simulink model "Linearization"  (R2022a)
settings: Solver=VariableStepAuto  StartTime=0.0  StopTime=100  RelTol=1e-3
undefined symbols (not defined in the file): Aactuator, ac, AeroCoeff, ControlAllocation, DUmax, DUmin, EngineTable, F, fcs, ft, g, hground, IC, kg, LandingGear, Light, LPmethod, m, MIL, Mode_deflection_aileron, Mode_deflection_elevator, Mode_deflection_rudder, Mode_deflection_TVC_y, Mode_deflection_TVC_z, N, Ninv_2nozzle, Ninv_no_nozzle, PIController, s, Sensor, slug, state0, sysID_DAQ, sysID_OBES, Umax_2nozzle, Umax_no_nozzle, Umin_2nozzle, Umin_no_nozzle, WMM2020
libraries: aerolibconvert2 x19, slpidlib x6, simulink x6, sharedutil x4, aerolibatmos2 x3, aerolibwind2 x3, aerolibbdyn x3, aerolibgravity2 x2, sharedtransform x1
(part 2 of 9)

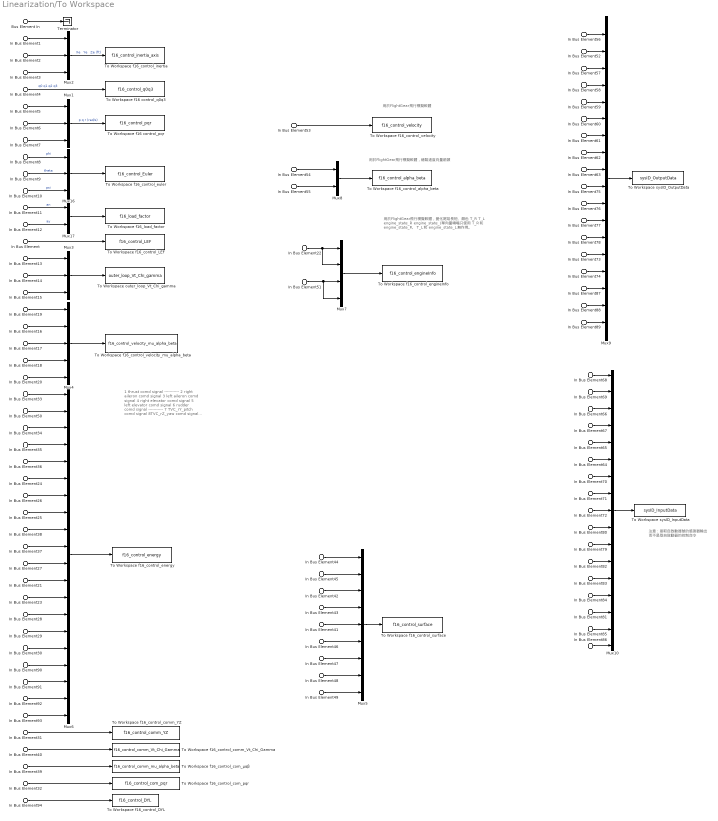
== system Linearization/To Workspace ==
  note: 1 thrust comd signal
      | -----------
      | 2 right aileron comd signal
      | 3 left aileron comd signal
      | 4 right elevator comd signal
      | 5 left elevator comd signal
      | 6 rudder comd signal
      | -----------
      | 7 TVC_rY_pitch comd signal
      | 8TVC_rZ_yaw comd signal
      | 9 TVC_lY_pitch comd signal
      | 10TVC_lZ_yaw comd signal
      |
      | 11 thrust signal
      | -----------
      | 12 right aileron signal
      | 13 left aileron signal
      | 14 right elevator signal
      | 15 left elevator signal
      | 16 rudder signal
      | -----------
      | 17 TVC_rY_pitch signal
      | 18 TVC_rZ_yaw signal
      | 19 TVC_lY_pitch signal
      | 20 TVC_lZ_yaw signal
  note: 用於FlightGear飛行模擬軟體
  note: 用於FlightGear飛行模擬軟體，繪製速度向量箭頭
  note: 用於FlightGear飛行模擬軟體，變化尾焰長短、顏色
      | T_R
      | T_L
      | engine_state_R
      | engine_state_L
      |
      | 單向量噴嘴只使用 T_R 和 engine_state_R。
      | T_L 和 engine_state_L 無作用。
  note: 注意：是取自致動器號的感測器輸出
      | 而不是取自致動器的控制命令
  In Bus Element1 : Inport  PortName=PlantData  Element=npos
  In Bus Element2 : Inport  PortName=PlantData  Element=epos
  In Bus Element3 : Inport  PortName=PlantData  Element=altitude
  In Bus Element4 : Inport  PortName=PlantData  Element=q0q1q2q3
  In Bus Element5 : Inport  PortName=PlantData  Element=p
  In Bus Element61 : Inport  PortName=PlantData  Element=p
  In Bus Element6 : Inport  PortName=PlantData  Element=q
  In Bus Element62 : Inport  PortName=PlantData  Element=q
  In Bus Element7 : Inport  PortName=PlantData  Element=r
  In Bus Element63 : Inport  PortName=PlantData  Element=r
  In Bus Element8 : Inport  PortName=PlantData  Element=phi
  In Bus Element58 : Inport  PortName=PlantData  Element=phi
  In Bus Element9 : Inport  PortName=PlantData  Element=theta
  In Bus Element59 : Inport  PortName=PlantData  Element=theta
  In Bus Element10 : Inport  PortName=PlantData  Element=psi
  In Bus Element60 : Inport  PortName=PlantData  Element=psi
  In Bus Element11 : Inport  PortName=PlantData  Element=an
  In Bus Element12 : Inport  PortName=PlantData  Element=ay
  In Bus Element : Inport  PortName=PlantData  Element=AeroActBus.LEF_deg
  In Bus Element80 : Inport  PortName=PlantData  Element=AeroActBus.LEF_deg
  In Bus Element30 : Inport  PortName=PlantData  Element=AeroActBus.Rudder_deg
  In Bus Element41 : Inport  PortName=PlantData  Element=AeroActBus.Rudder_deg
  In Bus Element65 : Inport  PortName=PlantData  Element=AeroActBus.Rudder_deg
  In Bus Element21 : Inport  PortName=PlantData  Element=AeroActBus.right Aileron_deg
  In Bus Element42 : Inport  PortName=PlantData  Element=AeroActBus.right Aileron_deg
  In Bus Element66 : Inport  PortName=PlantData  Element=AeroActBus.right Aileron_deg
  In Bus Element23 : Inport  PortName=PlantData  Element=AeroActBus.left Aileron_deg
  In Bus Element43 : Inport  PortName=PlantData  Element=AeroActBus.left Aileron_deg
  In Bus Element67 : Inport  PortName=PlantData  Element=AeroActBus.left Aileron_deg
  In Bus Element28 : Inport  PortName=PlantData  Element=AeroActBus.right Elevator_deg
  In Bus Element44 : Inport  PortName=PlantData  Element=AeroActBus.right Elevator_deg
  In Bus Element68 : Inport  PortName=PlantData  Element=AeroActBus.right Elevator_deg
  In Bus Element29 : Inport  PortName=PlantData  Element=AeroActBus.left Elevator_deg
  In Bus Element45 : Inport  PortName=PlantData  Element=AeroActBus.left Elevator_deg
  In Bus Element69 : Inport  PortName=PlantData  Element=AeroActBus.left Elevator_deg
  In Bus Element79 : Inport  PortName=PlantData  Element=AeroActBus.SB_deg
  In Bus Element{13,19,53,56} (4 alike) : Inport  PortName=PlantData  Element=Vt
  In Bus Element14 : Inport  PortName=PlantData  Element=chi
  In Bus Element88 : Inport  PortName=PlantData  Element=chi
  In Bus Element15 : Inport  PortName=PlantData  Element=gamma
  In Bus Element20 : Inport  PortName=PlantData  Element=gamma
  In Bus Element89 : Inport  PortName=PlantData  Element=gamma
  In Bus Element16 : Inport  PortName=PlantData  Element=alpha
  In Bus Element54 : Inport  PortName=PlantData  Element=alpha
  In Bus Element52 : Inport  PortName=PlantData  Element=alpha
  In Bus Element17 : Inport  PortName=PlantData  Element=beta
  In Bus Element55 : Inport  PortName=PlantData  Element=beta
  In Bus Element57 : Inport  PortName=PlantData  Element=beta
  In Bus Element18 : Inport  PortName=PlantData  Element=mu
  In Bus Element87 : Inport  PortName=PlantData  Element=mu
  In Bus Element33 : Inport  PortName=PlantData  Element=fadec_cmd.thrust
  In Bus Element25 : Inport  PortName=PlantData  Element=fadec_cmd.TVC_rz
  In Bus Element26 : Inport  PortName=PlantData  Element=fadec_cmd.TVC_ry
  In Bus Element37 : Inport  PortName=PlantData  Element=fadec_cmd.TVC_lz
  In Bus Element38 : Inport  PortName=PlantData  Element=fadec_cmd.TVC_ly
  In Bus Element24 : Inport  PortName=PlantData  Element=fcs_cmd.rudder
  In Bus Element34 : Inport  PortName=PlantData  Element=fcs_cmd.left aileron
  In Bus Element35 : Inport  PortName=PlantData  Element=fcs_cmd.right elevator
  In Bus Element36 : Inport  PortName=PlantData  Element=fcs_cmd.left elevator
  In Bus Element50 : Inport  PortName=PlantData  Element=fcs_cmd.right aileron
  In Bus Element27 : Inport  PortName=PlantData  Element=PropBus.T
  In Bus Element22 : Inport  PortName=PlantData  Element=PropBus.T
  In Bus Element51 : Inport  PortName=PlantData  Element=PropBus.engine_state
  In Bus Element82 : Inport  PortName=PlantData  Element=PropBus.Tx
  In Bus Element83 : Inport  PortName=PlantData  Element=PropBus.Ty
  In Bus Element84 : Inport  PortName=PlantData  Element=PropBus.Tz
  In Bus Element73 : Inport  PortName=PlantData  Element=ay_offset
  In Bus Element74 : Inport  PortName=PlantData  Element=az_offset
  In Bus Element75 : Inport  PortName=PlantData  Element=p_dot
  In Bus Element76 : Inport  PortName=PlantData  Element=q_dot
  In Bus Element77 : Inport  PortName=PlantData  Element=r_dot
  In Bus Element85 : Inport  PortName=PlantData  Element=f
  In Bus Element86 : Inport  PortName=PlantData  Element=N
  In Bus Element90 : Inport  PortName=PlantData  Element=PropActBus.TVC_ry_pitch_deg
  In Bus Element46 : Inport  PortName=PlantData  Element=PropActBus.TVC_ry_pitch_deg
  In Bus Element64 : Inport  PortName=PlantData  Element=PropActBus.TVC_ry_pitch_deg
  In Bus Element91 : Inport  PortName=PlantData  Element=PropActBus.TVC_rz_yaw_deg
  In Bus Element47 : Inport  PortName=PlantData  Element=PropActBus.TVC_rz_yaw_deg
  In Bus Element70 : Inport  PortName=PlantData  Element=PropActBus.TVC_rz_yaw_deg
  In Bus Element92 : Inport  PortName=PlantData  Element=PropActBus.TVC_ly_pitch_deg
  In Bus Element48 : Inport  PortName=PlantData  Element=PropActBus.TVC_ly_pitch_deg
  In Bus Element71 : Inport  PortName=PlantData  Element=PropActBus.TVC_ly_pitch_deg
  In Bus Element93 : Inport  PortName=PlantData  Element=PropActBus.TVC_lz_yaw_deg
  In Bus Element49 : Inport  PortName=PlantData  Element=PropActBus.TVC_lz_yaw_deg
  In Bus Element72 : Inport  PortName=PlantData  Element=PropActBus.TVC_lz_yaw_deg
  In Bus Element78 : Inport  PortName=PlantData  Element=ax_offset
  In Bus Element32 : Inport  PortName=PlantData  Element=LogDataBus.cmd_pqr
  In Bus Element39 : Inport  PortName=PlantData  Element=LogDataBus.cmd_mu_alpha_beta
  In Bus Element31 : Inport  PortName=PlantData  Element=LogDataBus.cmd_yz
  In Bus Element40 : Inport  PortName=PlantData  Element=LogDataBus.cmd_Vt_chi_gamma
  In Bus Element94 : Inport  PortName=PlantData  Element=LogDataBus.drag_sideForce_lift
  Bus Element In : Inport  Port=2  PortName=EnvData
  In Bus Element81 : Inport  Port=2  PortName=EnvData  Element=AirDensity
  Mux{1..3,16} (4 alike) : Mux  Inputs=3
  Mux10 : Mux  Inputs=17
  Mux17 : Mux  Inputs=2
  Mux4 : Mux  Inputs=5
  Mux5 : Mux  Inputs=9
  Mux6 : Mux  Inputs=20
  Mux7 : Mux
  Mux8 : Mux  Inputs=2
  Mux9 : Mux  Inputs=18
  Terminator : Terminator
  To Workspace f16 control_pqr : ToWorkspace  VariableName=f16_control_pqr  SaveFormat=Timeseries  SampleTime=-1
  To Workspace f16 control_q0q3 : ToWorkspace  VariableName=f16_control_q0q3  SaveFormat=Timeseries  SampleTime=-1
  To Workspace f16_control_DYL : ToWorkspace  VariableName=f16_control_DYL  SaveFormat=Timeseries  SampleTime=-1
  To Workspace f16_control_LEF : ToWorkspace  VariableName=f16_control_LEF  SaveFormat=Timeseries  SampleTime=-1
  To Workspace f16_control_alpha_beta : ToWorkspace  VariableName=f16_control_alpha_beta  SaveFormat=Timeseries  SampleTime=-1
  To Workspace f16_control_com_pqr : ToWorkspace  VariableName=f16_control_com_pqr  SaveFormat=Timeseries  SampleTime=-1
  To Workspace f16_control_com_μαβ : ToWorkspace  VariableName=f16_control_comm_mu_alpha_beta  SaveFormat=Timeseries  SampleTime=-1
  To Workspace f16_control_comm_Vt_Chi_Gamma : ToWorkspace  VariableName=f16_control_comm_Vt_Chi_Gamma  SaveFormat=Timeseries  SampleTime=-1
  To Workspace f16_control_comm_YZ : ToWorkspace  VariableName=f16_control_comm_YZ  SaveFormat=Timeseries  SampleTime=-1
  To Workspace f16_control_energy : ToWorkspace  VariableName=f16_control_energy  SaveFormat=Timeseries  SampleTime=-1
  To Workspace f16_control_engineInfo : ToWorkspace  VariableName=f16_control_engineInfo  SaveFormat=Timeseries  SampleTime=-1
  To Workspace f16_control_euler : ToWorkspace  VariableName=f16_control_Euler  SaveFormat=Timeseries  SampleTime=-1
  To Workspace f16_control_inertia : ToWorkspace  VariableName=f16_control_inertia_axis  SaveFormat=Timeseries  SampleTime=-1
      settings: Save2DSignal=2-D array (concatenate along first dimension)
  To Workspace f16_control_surface : ToWorkspace  VariableName=f16_control_surface  SaveFormat=Timeseries  SampleTime=-1
  To Workspace f16_control_velocity : ToWorkspace  VariableName=f16_control_velocity  SaveFormat=Timeseries  SampleTime=-1
  To Workspace f16_control_velocity_mu_alpha_beta : ToWorkspace  VariableName=f16_control_velocity_mu_alpha_beta  SaveFormat=Timeseries  SampleTime=-1
  To Workspace f16_load_factor : ToWorkspace  VariableName=f16_load_factor  SaveFormat=Timeseries  SampleTime=-1
  To Workspace outer_loop_Vt_Chi_gamma : ToWorkspace  VariableName=outer_loop_Vt_Chi_gamma  SaveFormat=Timeseries  SampleTime=-1
  To Workspace sysID_InputData : ToWorkspace  VariableName=sysID_InputData  SaveFormat=Timeseries  SampleTime=sysID_DAQ.sampleTime
  To Workspace sysID_OutputData : ToWorkspace  VariableName=sysID_OutputData  SaveFormat=Timeseries  SampleTime=sysID_DAQ.sampleTime
  wires:
  Mux2/1 -> To Workspace f16_control_inertia/1  "Xe   Ye   Ze (ft)"
  Mux16/1 -> To Workspace f16_control_euler/1
  In Bus Element9/1 -> Mux16/2  "theta"
  In Bus Element10/1 -> Mux16/3  "psi"
  In Bus Element4/1 -> To Workspace f16 control_q0q3/1  "q0 q1 q2 q3"
  In Bus Element11/1 -> Mux17/1  "an"
  In Bus Element8/1 -> Mux16/1  "phi"
  Mux17/1 -> To Workspace f16_load_factor/1
  In Bus Element12/1 -> Mux17/2  "ay"
  Mux1/1 -> To Workspace f16 control_pqr/1  "p q r (rad/s)"
  In Bus Element5/1 -> Mux1/1
  In Bus Element6/1 -> Mux1/2
  In Bus Element7/1 -> Mux1/3
  In Bus Element1/1 -> Mux2/1
  In Bus Element2/1 -> Mux2/2
  In Bus Element3/1 -> Mux2/3
  In Bus Element/1 -> To Workspace f16_control_LEF/1
  In Bus Element13/1 -> Mux3/1
  In Bus Element14/1 -> Mux3/2
  In Bus Element15/1 -> Mux3/3
  Mux3/1 -> To Workspace outer_loop_Vt_Chi_gamma/1
  In Bus Element19/1 -> Mux4/1
  In Bus Element16/1 -> Mux4/2
  In Bus Element17/1 -> Mux4/3
  In Bus Element18/1 -> Mux4/4
  In Bus Element20/1 -> Mux4/5
  Mux4/1 -> To Workspace f16_control_velocity_mu_alpha_beta/1
  Mux6/1 -> To Workspace f16_control_energy/1
  Bus Element In/1 -> Terminator/1
  In Bus Element33/1 -> Mux6/1
  In Bus Element50/1 -> Mux6/2
  In Bus Element34/1 -> Mux6/3
  In Bus Element35/1 -> Mux6/4
  In Bus Element36/1 -> Mux6/5
  In Bus Element24/1 -> Mux6/6
  In Bus Element27/1 -> Mux6/11
  In Bus Element21/1 -> Mux6/12
  In Bus Element23/1 -> Mux6/13
  In Bus Element28/1 -> Mux6/14
  In Bus Element29/1 -> Mux6/15
  In Bus Element30/1 -> Mux6/16
  In Bus Element90/1 -> Mux6/17
  In Bus Element91/1 -> Mux6/18
  In Bus Element92/1 -> Mux6/19
  In Bus Element93/1 -> Mux6/20
  In Bus Element41/1 -> Mux5/5
  In Bus Element47/1 -> Mux5/7
  In Bus Element49/1 -> Mux5/9
  In Bus Element48/1 -> Mux5/8
  In Bus Element46/1 -> Mux5/6
  In Bus Element44/1 -> Mux5/1
  In Bus Element45/1 -> Mux5/2
  In Bus Element42/1 -> Mux5/3
  In Bus Element43/1 -> Mux5/4
  Mux5/1 -> To Workspace f16_control_surface/1
  In Bus Element26/1 -> Mux6/7
  In Bus Element25/1 -> Mux6/8
  In Bus Element38/1 -> Mux6/9
  In Bus Element37/1 -> Mux6/10
  Mux8/1 -> To Workspace f16_control_alpha_beta/1
  In Bus Element53/1 -> To Workspace f16_control_velocity/1
  In Bus Element55/1 -> Mux8/2
  In Bus Element54/1 -> Mux8/1
  Mux7/1 -> To Workspace f16_control_engineInfo/1
  In Bus Element22/1 -> Mux7/2, Mux7/1
  In Bus Element51/1 -> Mux7/4, Mux7/3
  In Bus Element78/1 -> Mux9/13
  In Bus Element65/1 -> Mux10/5
  In Bus Element75/1 -> Mux9/10
  In Bus Element80/1 -> Mux10/10
  In Bus Element52/1 -> Mux9/2
  In Bus Element79/1 -> Mux10/11
  In Bus Element59/1 -> Mux9/5
  In Bus Element62/1 -> Mux9/8
  In Bus Element83/1 -> Mux10/13
  In Bus Element73/1 -> Mux9/14
  In Bus Element71/1 -> Mux10/8
  In Bus Element60/1 -> Mux9/6
  In Bus Element61/1 -> Mux9/7
  In Bus Element68/1 -> Mux10/1
  In Bus Element77/1 -> Mux9/12
  In Bus Element66/1 -> Mux10/3
  In Bus Element72/1 -> Mux10/9
  In Bus Element69/1 -> Mux10/2
  In Bus Element70/1 -> Mux10/7
  In Bus Element63/1 -> Mux9/9
  In Bus Element58/1 -> Mux9/4
  In Bus Element57/1 -> Mux9/3
  In Bus Element86/1 -> Mux10/17
  In Bus Element67/1 -> Mux10/4
  In Bus Element88/1 -> Mux9/17
  In Bus Element85/1 -> Mux10/16
  In Bus Element76/1 -> Mux9/11
  In Bus Element84/1 -> Mux10/14
  In Bus Element81/1 -> Mux10/15
  In Bus Element82/1 -> Mux10/12
  In Bus Element87/1 -> Mux9/16
  In Bus Element74/1 -> Mux9/15
  In Bus Element89/1 -> Mux9/18
  In Bus Element64/1 -> Mux10/6
  Mux10/1 -> To Workspace sysID_InputData/1
  In Bus Element56/1 -> Mux9/1
  Mux9/1 -> To Workspace sysID_OutputData/1
  In Bus Element32/1 -> To Workspace f16_control_com_pqr/1
  In Bus Element39/1 -> To Workspace f16_control_com_μαβ/1
  In Bus Element31/1 -> To Workspace f16_control_comm_YZ/1
  In Bus Element40/1 -> To Workspace f16_control_comm_Vt_Chi_Gamma/1
  In Bus Element94/1 -> To Workspace f16_control_DYL/1

== system Linearization/Vehicle ==
  note: 重心高度只取體軸z，因假設機腹朝下。
      | 更正確做法是要乘上旋轉座標DCM_eb
  note: 為了避免無謂計算，縮短模擬時間，
      | 只有在「飛機重心靠近地面」並且「起落架放下」的情況，
      | 才開始計算地面反作用力
  note: 設定Port dimensions=3
  note: 攻角 $\alpha$ 限制 -20 ~ 90度
      | 側滑角 $\beta$ 限制 -30 ~ 30 度
      | 馬赫數限制 0.1 ~ 0.6 度
  note: Tx
      | Ty
      | Tz
      | ---
      | Mx_T
      | My_T
      | Mz_T
  note: 高度限制 0 ~ 50000 ft
      | 馬赫數限制 0 ~ 1 馬赫
  note: f
      | 0
      | N
  note: TODO: 改成local變數
      | 或者應該新增為OBM機載模型!?
      | 或者空中NDI跟地面NDI控制器分離!?
  note: Nonlinear Model
  fadec_cmd : Inport
  fcs_cmd : Inport  Port=2
  " SB_deg" : Inport  Port=3
  LG_cmd : Inport  Port=4
  Bus Element In{,1..3} (4 alike) : Inport  Port=5  PortName=EnvData
  In Bus Element : Inport  Port=5  PortName=EnvData  Element=g
  LogDataBus : Inport  Port=6
  6DOF (Quaternion) : Subsystem
  Actuators (no roll off)1 : Subsystem  Commented=on
  Aerodynamics : Subsystem
  Bus Selector : BusSelector  OutputSignals=altitude
  Compare To Constant : simulink/Logic and Bit Operations/Compare To Constant  relop=>=  const=-30  OutDataTypeStr=boolean
  Demux2 : Demux  Outputs=[3, 3]
  Demux3 : Demux  Outputs=3
  Demux4 : Demux  Outputs=[3, 3]
  Gravity Force : Subsystem
  LandingGear GroundReaction : Subsystem
  Logical Operator : Logic  AllPortsSameDT=off  OutDataTypeStr=boolean
  Logical Operator1 : Logic  Operator=OR  Inputs=1  AllPortsSameDT=off  OutDataTypeStr=boolean
  ModelBus : BusCreator  Inputs=39
  Propulsion : Subsystem  Commented=on
  Propulsion(two_nozzles) : Subsystem
  Selector : Selector  InputPortWidth=3  IndexOptions=Index vector (dialog)  Indices=3  OutputSizes=1
  Selector1 : Selector  InputPortWidth=6  IndexOptions=Index vector (dialog)  Indices=[1 2 3]  OutputSizes=1
  Selector2 : Selector  InputPortWidth=6  IndexOptions=Index vector (dialog)  Indices=[1 2 3]  OutputSizes=1
  Signal Specification : SignalSpecification  Dimensions=3
  Sum : Sum  Inputs=||+++
  Sum1 : Sum  Inputs=++|
  Terminator3 : Terminator
  PlantData : Outport
  tag scope: LGxyz=global
  wires:
  " SB_deg"/1 -> Aerodynamics/2(" SB (deg)")
  Aerodynamics/1(FM) -> Sum/2, 6DOF (Quaternion)/4(AeroFM)
  Aerodynamics/2(ActSensor_Out) -> [AeroActBus]
  Propulsion(two_nozzles)/1(FM) -> Selector2/1, Sum/1
  fcs_cmd/1 -> Aerodynamics/1(fcs_cmd), [fcs_cmd]  "fcs_cmd"
  fadec_cmd/1 -> Propulsion(two_nozzles)/1(fadec_cmd), [fadec_cmd]  "fadec_cmd"
  Propulsion(two_nozzles)/2(ActSensor_Out) -> [PropActBus]
  Propulsion(two_nozzles)/3(PropData) -> [PropBus]
  Sum/1 -> Demux4/1
  Sum1/1 -> 6DOF (Quaternion)/1(Fxyz)
  Bus Element In/1 -> Aerodynamics/3(EnvData)
  Bus Element In1/1 -> Propulsion(two_nozzles)/2(EnvData)
  LandingGear GroundReaction/1(FM) -> Demux2/1, Sum/3, Selector1/1
  Selector1/1 -> 6DOF (Quaternion)/5(LGxyz)
  Demux2/1 -> [LGxyz]
  Demux2/2 -> Terminator3/1
  Signal Specification/1 -> Logical Operator1/1, LandingGear GroundReaction/1(LG_cmd)
  LandingGear GroundReaction/2(LGData) -> [LGBus]
  Logical Operator/1 -> LandingGear GroundReaction/Enable
  Compare To Constant/1 -> Logical Operator/1
  Bus Selector/1 -> Compare To Constant/1  "<altitude>"
  Logical Operator1/1 -> Logical Operator/2
  LG_cmd/1 -> Signal Specification/1
  Gravity Force/1(Fgrav) -> Sum1/1
  Demux4/1 -> Sum1/2
  Bus Element In3/1 -> Gravity Force/2(EnvData)
  Bus Element In2/1 -> LandingGear GroundReaction/2(EnvData)
  In Bus Element/1 -> Selector/1
  [PropActBus] -> ModelBus/35  "PropActBus"
  Demux3/2 -> ModelBus/31
  6DOF (Quaternion)/22(ay_cg) -> ModelBus/22  "ay_cg"
  Demux3/3 -> ModelBus/32  "N"
  Demux3/1 -> ModelBus/30  "f"
  6DOF (Quaternion)/2(DCM_eb) -> ModelBus/2  "DCM_eb"
  6DOF (Quaternion)/18(r) -> ModelBus/18  "r"
  6DOF (Quaternion)/8(theta) -> ModelBus/8  "theta"
  [fadec_cmd] -> ModelBus/36
  6DOF (Quaternion)/21(ax_cg) -> ModelBus/21  "ax_cg"
  [LGBus] -> ModelBus/38  "LGBus"
  6DOF (Quaternion)/3(npos) -> ModelBus/3  "npos"
  6DOF (Quaternion)/10(mu) -> ModelBus/10  "mu"
  [fcs_cmd] -> ModelBus/37
  [AeroActBus] -> ModelBus/33  "AeroActBus"
  6DOF (Quaternion)/16(p) -> ModelBus/16  "p"
  6DOF (Quaternion)/17(q) -> ModelBus/17  "q"
  6DOF (Quaternion)/13(Vt) -> ModelBus/13  "Vt"
  6DOF (Quaternion)/29(r_dot) -> ModelBus/29  "r_dot"
  6DOF (Quaternion)/24(ax_offset) -> ModelBus/24  "ax_offset"
  6DOF (Quaternion)/28(q_dot) -> ModelBus/28  "q_dot"
  6DOF (Quaternion)/19(an) -> ModelBus/19  "an"
  6DOF (Quaternion)/20(ay) -> ModelBus/20  "ay"
  6DOF (Quaternion)/6(q0q1q2q3) -> ModelBus/6  "q0q1q2q3"
  6DOF (Quaternion)/11(gamma) -> ModelBus/11  "gamma"
  6DOF (Quaternion)/27(p_dot) -> ModelBus/27  "p_dot"
  6DOF (Quaternion)/9(psi) -> ModelBus/9  "psi"
  6DOF (Quaternion)/5(altitude) -> ModelBus/5  "altitude"
  6DOF (Quaternion)/7(phi) -> ModelBus/7  "phi"
  6DOF (Quaternion)/14(alpha) -> ModelBus/14  "alpha"
  6DOF (Quaternion)/4(epos) -> ModelBus/4  "epos"
  6DOF (Quaternion)/15(beta) -> ModelBus/15  "beta"
  6DOF (Quaternion)/1(DCM_be) -> Gravity Force/1(DCM_be), ModelBus/1  "DCM_be"
  6DOF (Quaternion)/23(az_cg) -> ModelBus/23  "az_cg"
  [LGxyz] -> Demux3/1
  ModelBus/1 -> LandingGear GroundReaction/3(PlantData), Bus Selector/1, Propulsion(two_nozzles)/3(PlantData), Aerodynamics/4(PlantData), PlantData/1  "PlantData"
  6DOF (Quaternion)/25(ay_offset) -> ModelBus/25  "ay_offset"
  6DOF (Quaternion)/12(chi) -> ModelBus/12  "chi"
  [PropBus] -> ModelBus/34  "PropBus"
  6DOF (Quaternion)/26(az_offset) -> ModelBus/26  "az_offset"
  Demux4/2 -> 6DOF (Quaternion)/2(Mxyz)
  Selector2/1 -> 6DOF (Quaternion)/3(Txyz)
  Selector/1 -> 6DOF (Quaternion)/6(gravity)
  LogDataBus/1 -> ModelBus/39  "LogDataBus"

== system Linearization/pqr NDI Controller ==
  note: $\hat{L}, \hat{M}, \hat{N}$
  note: 【有向量噴嘴控制】
      | (註：有/無向量噴嘴的差異之處在於 "粉紅色模塊" 的內容)
  note: 1  gp_dra1
      |     gp_dla1
      |     gp_dre1
      |     gp_dle1
      |     gp_dr1
      |     gp_dra2
      |     gp_dla2
      |     gp_dre2
      |     gp_dle2
      |     gp_dr2
      |
      | 11 gq_dra
      |      gq_dla
      |      gq_dre
      |      gq_dle
      |
      | 15 gr_dra1
      |      gr_dla1
      |      gr_dre1
      |      gr_dle1
      |      gr_dr1
      |      gr_dra2
      |      gr_dla2
      |      gr_dre2
      |      gr_dle2
      |      gr_dr2
  note: $g_1 {\left({\overset{-}{x} }_1 \right)}={\left[\begin{array}{ccccccccc} g_{p_{\delta_{ra} } } & g_{p_{\delta_{la} } } & g_{p_{\delta_{re} } } & g_{p_{\delta_{le} } } & g_{p_{\delta_r } } & g_{p_{\delta_{ry} } } & g_{p_{\delta_{rz} } } & g_{p_{\delta_{ly} } } & g_{p_{\delta_{lz} } } \\ g_{q_{\delta_{ra} } } & g_{q_{\delta_{la} } } & g_{q_{\delta_{re} } } & g_{q_{\delta_{le} } } & 0 & g_{q_{\delta_{ry} } } & 0 & g_{q_{\delta_{ly} } } & 0 \\ g_{r_{\delta_{ra} } } & g_{r_{\delta_{la} } } & g_{r_{\delta_{re} } } & g_{r_{\delta_{le} } } & g_{r_{\delta_r } } & g_{r_{\delta_{ry} } } & g_{r_{\delta_{rz} } } & g_{r_{\delta_{ly} } } & g_{r_{\delta_{lz} } } \end{array}\right]}$
  note: 選擇偏轉模式
  coef M : Inport
  control g : Inport  Port=2
  pqr dot desire : Inport  Port=3
  p q r : Inport  Port=4
  In Bus Element : Inport  Port=5  PortName=PlantData  Element=PropBus.T
  In Bus Element12 : Inport  Port=5  PortName=PlantData  Element=alpha
  In Bus Element13 : Inport  Port=5  PortName=PlantData  Element=Vt
  In Bus Element14 : Inport  Port=5  PortName=PlantData  Element=altitude
  " f1" : MATLAB Function  TreatAsAtomicUnit=on
  Constant : Constant  Value=0
  Constant1 : Constant  Value=N
  Control Allocation : Subsystem
  Demux : Demux  Outputs=9
  Ix(slug*ft^2)1 : Constant  Value=ac.Ix
  Ixz(slug*ft^2)1 : Constant  Value=ac.Ixz
  Iy(slug*ft^2)1 : Constant  Value=ac.Iy
  Iz(slug*ft^2)1 : Constant  Value=ac.Iz
  MakeINMAT : Subsystem
  Mode_deflection : Subsystem
  Sum : Sum  Inputs=+-|
  To Workspace3 : ToWorkspace  VariableName=upast  SaveFormat=Timeseries  SampleTime=-1
  Unit Delay : UnitDelay  InitialCondition=[0 0 0 0 0 0 0 0 0]  SampleTime=fcs.Ts  HasFrameUpgradeWarning=on
  control matrix g1 : Subsystem
  left_rudder : Terminator
  "TVC_ry " : Outport  VectorParamsAs1DForOutWhenUnconnected=off
  TVC_rz : Outport  Port=2  VectorParamsAs1DForOutWhenUnconnected=off
  "TVC_ly " : Outport  Port=3  VectorParamsAs1DForOutWhenUnconnected=off
  "TVC_lz " : Outport  Port=4  VectorParamsAs1DForOutWhenUnconnected=off
  right_aileron : Outport  Port=5  VectorParamsAs1DForOutWhenUnconnected=off
  left_aileron : Outport  Port=6  VectorParamsAs1DForOutWhenUnconnected=off
  right_elevator : Outport  Port=7  VectorParamsAs1DForOutWhenUnconnected=off
  left_elevator : Outport  Port=8  VectorParamsAs1DForOutWhenUnconnected=off
  rudder : Outport  Port=9  VectorParamsAs1DForOutWhenUnconnected=off
  wires:
  coef M/1 -> " f1"/1(moments)
  p q r/1 -> " f1"/2(pqr)
  " f1"/1(f1) -> Sum/2
  pqr dot desire/1 -> Sum/1
  In Bus Element/1 -> control matrix g1/2(Thrust T)
  control g/1 -> control matrix g1/1(coef g)
  Iy(slug*ft^2)1/1 -> " f1"/4(Iy)
  Ix(slug*ft^2)1/1 -> " f1"/3(Ix)
  Iz(slug*ft^2)1/1 -> " f1"/5(Iz)
  Ixz(slug*ft^2)1/1 -> " f1"/6(Ixz)
  MakeINMAT/1(IN_MAT) -> Control Allocation/1(IN_MAT1)
  Sum/1 -> Control Allocation/5(y_bar), MakeINMAT/1(f1)
  control matrix g1/1(g1) -> MakeINMAT/2(g1), Control Allocation/6(g1)
  Control Allocation/1(Du) -> Unit Delay/1, To Workspace3/1, Demux/1
  Unit Delay/1 -> MakeINMAT/3(In3)
  In Bus Element12/1 -> Control Allocation/2(Input)
  In Bus Element13/1 -> Control Allocation/3(Input1)
  In Bus Element14/1 -> Control Allocation/4(Input2)
  Constant/1 -> Mode_deflection/6(dlr)
  Constant1/1 -> Control Allocation/7(N)
  Demux/9 -> Mode_deflection/10(dlz)
  Demux/1 -> Mode_deflection/1(dra)
  Demux/2 -> Mode_deflection/2(dla)
  Demux/5 -> Mode_deflection/5(drr)
  Demux/4 -> Mode_deflection/4(dle)
  Demux/8 -> Mode_deflection/9(dly)
  Demux/6 -> Mode_deflection/7(dry)
  Demux/3 -> Mode_deflection/3(dre)
  Demux/7 -> Mode_deflection/8(drz)
  Mode_deflection/9("TVC_ly ") -> "TVC_ly "/1
  Mode_deflection/10("TVC_lz ") -> "TVC_lz "/1
  Mode_deflection/7("TVC_ry ") -> "TVC_ry "/1
  Mode_deflection/8(TVC_rz) -> TVC_rz/1
  Mode_deflection/2(left_aileron) -> left_aileron/1
  Mode_deflection/4(left_elevator) -> left_elevator/1
  Mode_deflection/6(left_rudder) -> left_rudder/1
  Mode_deflection/1(right_aileron) -> right_aileron/1
  Mode_deflection/3(right_elevator) -> right_elevator/1
  Mode_deflection/5(rudder) -> rudder/1

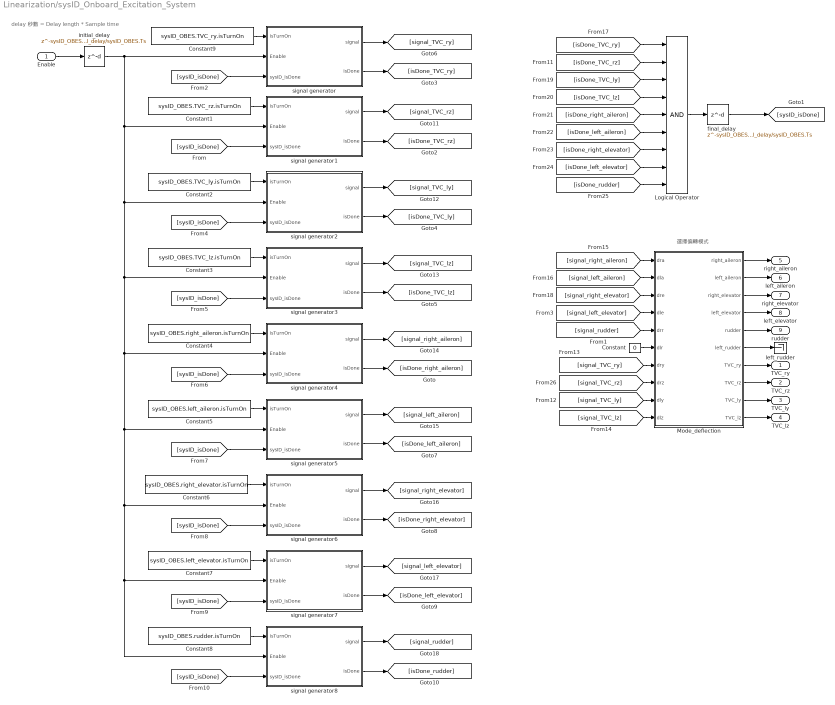
== system Linearization/sysID_Onboard_Excitation_System ==
  note: delay 秒數 = Delay length * Sample time
  note: 選擇偏轉模式
  Enable : Inport
  Constant : Constant  Value=0
  Constant1 : Constant  Value=sysID_OBES.TVC_rz.isTurnOn
  Constant2 : Constant  Value=sysID_OBES.TVC_ly.isTurnOn
  Constant3 : Constant  Value=sysID_OBES.TVC_lz.isTurnOn
  Constant4 : Constant  Value=sysID_OBES.right_aileron.isTurnOn
  Constant5 : Constant  Value=sysID_OBES.left_aileron.isTurnOn
  Constant6 : Constant  Value=sysID_OBES.right_elevator.isTurnOn
  Constant7 : Constant  Value=sysID_OBES.left_elevator.isTurnOn
  Constant8 : Constant  Value=sysID_OBES.rudder.isTurnOn
  Constant9 : Constant  Value=sysID_OBES.TVC_ry.isTurnOn
  Logical Operator : Logic  Inputs=9  AllPortsSameDT=off  OutDataTypeStr=boolean
  Mode_deflection : Subsystem
  final_delay : Delay  DelayLength=sysID_OBES.final_delay/sysID_OBES.Ts  SampleTime=sysID_OBES.Ts
  initial_delay : Delay  DelayLength=sysID_OBES.initial_delay/sysID_OBES.Ts  SampleTime=sysID_OBES.Ts
  left_rudder : Terminator
  signal generator : Subsystem  TreatAsAtomicUnit=on
  signal generator1 : Subsystem  TreatAsAtomicUnit=on
  signal generator2 : Subsystem  TreatAsAtomicUnit=on
  signal generator3 : Subsystem  TreatAsAtomicUnit=on
  signal generator4 : Subsystem  TreatAsAtomicUnit=on
  signal generator5 : Subsystem  TreatAsAtomicUnit=on
  signal generator6 : Subsystem  TreatAsAtomicUnit=on
  signal generator7 : Subsystem  TreatAsAtomicUnit=on
  signal generator8 : Subsystem  TreatAsAtomicUnit=on
  TVC_ry : Outport
  TVC_rz : Outport  Port=2
  TVC_ly : Outport  Port=3
  TVC_lz : Outport  Port=4
  right_aileron : Outport  Port=5
  left_aileron : Outport  Port=6
  right_elevator : Outport  Port=7
  left_elevator : Outport  Port=8
  rudder : Outport  Port=9
  wires:
  Logical Operator/1 -> final_delay/1
  final_delay/1 -> [sysID_isDone]
  signal generator1/2(isDone) -> [isDone_TVC_rz]
  [sysID_isDone] -> signal generator1/3(sysID_isDone)
  Enable/1 -> initial_delay/1
  signal generator/2(isDone) -> [isDone_TVC_ry]
  [sysID_isDone] -> signal generator/3(sysID_isDone)
  signal generator2/2(isDone) -> [isDone_TVC_ly]
  [sysID_isDone] -> signal generator2/3(sysID_isDone)
  signal generator3/2(isDone) -> [isDone_TVC_lz]
  [sysID_isDone] -> signal generator3/3(sysID_isDone)
  signal generator4/2(isDone) -> [isDone_right_aileron]
  [sysID_isDone] -> signal generator4/3(sysID_isDone)
  signal generator5/2(isDone) -> [isDone_left_aileron]
  [sysID_isDone] -> signal generator5/3(sysID_isDone)
  [sysID_isDone] -> signal generator6/3(sysID_isDone)
  signal generator6/2(isDone) -> [isDone_right_elevator]
  [sysID_isDone] -> signal generator7/3(sysID_isDone)
  signal generator7/2(isDone) -> [isDone_left_elevator]
  [sysID_isDone] -> signal generator8/3(sysID_isDone)
  initial_delay/1 -> signal generator1/2(Enable), signal generator2/2(Enable), signal generator3/2(Enable), signal generator4/2(Enable), signal generator5/2(Enable), signal generator6/2(Enable), signal generator8/2(Enable), signal generator7/2(Enable), signal generator/2(Enable)
  signal generator8/2(isDone) -> [isDone_rudder]
  Constant1/1 -> signal generator1/1(isTurnOn)
  Constant2/1 -> signal generator2/1(isTurnOn)
  Constant3/1 -> signal generator3/1(isTurnOn)
  Constant4/1 -> signal generator4/1(isTurnOn)
  Constant5/1 -> signal generator5/1(isTurnOn)
  Constant6/1 -> signal generator6/1(isTurnOn)
  Constant7/1 -> signal generator7/1(isTurnOn)
  Constant8/1 -> signal generator8/1(isTurnOn)
  Constant/1 -> Mode_deflection/6(dlr)
  Constant9/1 -> signal generator/1(isTurnOn)
  [isDone_TVC_ly] -> Logical Operator/3
  [isDone_TVC_lz] -> Logical Operator/4
  [isDone_right_aileron] -> Logical Operator/5
  [isDone_left_aileron] -> Logical Operator/6
  [isDone_right_elevator] -> Logical Operator/7
  [isDone_left_elevator] -> Logical Operator/8
  [signal_TVC_ry] -> Mode_deflection/7(dry)
  [isDone_rudder] -> Logical Operator/9
  [signal_TVC_ly] -> Mode_deflection/9(dly)
  [isDone_TVC_ry] -> Logical Operator/1
  [signal_TVC_lz] -> Mode_deflection/10(dlz)
  [signal_right_aileron] -> Mode_deflection/1(dra)
  [signal_left_aileron] -> Mode_deflection/2(dla)
  [signal_right_elevator] -> Mode_deflection/3(dre)
  [signal_left_elevator] -> Mode_deflection/4(dle)
  [signal_rudder] -> Mode_deflection/5(drr)
  [signal_TVC_rz] -> Mode_deflection/8(drz)
  [isDone_TVC_rz] -> Logical Operator/2
  Mode_deflection/9("TVC_ly ") -> TVC_ly/1
  Mode_deflection/10("TVC_lz ") -> TVC_lz/1
  Mode_deflection/7("TVC_ry ") -> TVC_ry/1
  Mode_deflection/8(TVC_rz) -> TVC_rz/1
  Mode_deflection/2(left_aileron) -> left_aileron/1
  Mode_deflection/4(left_elevator) -> left_elevator/1
  Mode_deflection/6(left_rudder) -> left_rudder/1
  Mode_deflection/1(right_aileron) -> right_aileron/1
  Mode_deflection/3(right_elevator) -> right_elevator/1
  Mode_deflection/5(rudder) -> rudder/1
  signal generator1/1(signal) -> [signal_TVC_rz]
  signal generator2/1(signal) -> [signal_TVC_ly]
  signal generator3/1(signal) -> [signal_TVC_lz]
  signal generator4/1(signal) -> [signal_right_aileron]
  signal generator5/1(signal) -> [signal_left_aileron]
  signal generator6/1(signal) -> [signal_right_elevator]
  signal generator7/1(signal) -> [signal_left_elevator]
  signal generator8/1(signal) -> [signal_rudder]
  signal generator/1(signal) -> [signal_TVC_ry]

== system Linearization/μαβ NDI Controller ==
  aero F : Inport
  μαβ dot desire : Inport  Port=2
  LGxyz : Inport  Port=3
  gravity : Inport  Port=4
  In Bus Element : Inport  Port=5  PortName=PlantData  Element=PropBus.T
  In Bus Element1 : Inport  Port=5  PortName=PlantData  Element=chi
  In Bus Element2 : Inport  Port=6  PortName=AirData  Element=alpha
  In Bus Element4 : Inport  Port=6  PortName=AirData  Element=alpha
  In Bus Element3 : Inport  Port=6  PortName=AirData  Element=beta
  In Bus Element5 : Inport  Port=6  PortName=AirData  Element=beta
  In Bus Element6 : Inport  Port=6  PortName=AirData  Element=mu
  In Bus Element7 : Inport  Port=6  PortName=AirData  Element=Vt
  In Bus Element8 : Inport  Port=6  PortName=AirData  Element=gamma
  Mux : Mux  Inputs=5
  Sum : Sum  Inputs=+-|
  attitude NDI : MATLAB Function  TreatAsAtomicUnit=on
  command matrix : Subsystem
  f2 : Subsystem
  pc : Outport  VectorParamsAs1DForOutWhenUnconnected=off
  qc : Outport  Port=2  VectorParamsAs1DForOutWhenUnconnected=off
  rc : Outport  Port=3  VectorParamsAs1DForOutWhenUnconnected=off
  D : Outport  Port=4  VectorParamsAs1DForOutWhenUnconnected=off
  Y : Outport  Port=5  VectorParamsAs1DForOutWhenUnconnected=off
  L : Outport  Port=6  VectorParamsAs1DForOutWhenUnconnected=off
  wires:
  f2/1(f2) -> Sum/2
  μαβ dot desire/1 -> Sum/1
  Sum/1 -> attitude NDI/1(y_bar)
  attitude NDI/1(p_c) -> pc/1
  attitude NDI/2(q_c) -> qc/1
  attitude NDI/3(r_c) -> rc/1
  command matrix/1(g2) -> attitude NDI/2(g2)
  Mux/1 -> f2/1(aero V)  "V, α, β, μ, γ"
  In Bus Element/1 -> f2/4(Thrust)
  aero F/1 -> f2/2(X,Y,Z)
  f2/2(D) -> D/1
  f2/3(Y) -> Y/1
  f2/4(L) -> L/1
  gravity/1 -> f2/3(gravity)
  In Bus Element2/1 -> command matrix/1(α)
  In Bus Element3/1 -> command matrix/2(β)
  In Bus Element5/1 -> Mux/3
  In Bus Element4/1 -> Mux/2
  In Bus Element6/1 -> Mux/4
  In Bus Element7/1 -> Mux/1
  In Bus Element8/1 -> Mux/5
  LGxyz/1 -> f2/5(LGxyz)
  In Bus Element1/1 -> f2/6(chi)

== system Linearization/Aerodynamic1/Creating    qbar // ps ==
  h (ft) : Inport
  Vt (ft/s) : Inport  Port=2
  Constant2 : Constant
  Constant3 : Constant  Value=390
  Constant6 : Constant  Value=4.14
  Math Function : Math  Operator=pow  SignedPower=on
  Math Function1 : Math  Operator=square  SignedPower=on
  Product : Product  Inputs=/*  InputSameDT=on  SaturateOnIntegerOverflow=on  OutDataTypeStr=Inherit: Same as first input
  Product5 : Product  Inputs=**  InputSameDT=on  SaturateOnIntegerOverflow=on  OutDataTypeStr=Inherit: Same as first input
  Product6 : Product  Inputs=**  InputSameDT=on  SaturateOnIntegerOverflow=on  OutDataTypeStr=Inherit: Same as first input
  Sum3 : Sum  Inputs=+-|  InputSameDT=on  SaturateOnIntegerOverflow=on  OutDataTypeStr=Inherit: Same as first input
  Switch : Switch  Threshold=35000
  r2d2 : Gain  Gain=0.703e-5  SaturateOnIntegerOverflow=on  OutDataTypeStr=Inherit: Same as input  ParamDataTypeStr=Inherit: Same as input
  r2d3 : Gain  Gain=519  SaturateOnIntegerOverflow=on  OutDataTypeStr=Inherit: Same as input  ParamDataTypeStr=Inherit: Same as input
  r2d4 : Gain  Gain=0.5  SaturateOnIntegerOverflow=on  OutDataTypeStr=Inherit: Same as input  ParamDataTypeStr=Inherit: Same as input
  r2d5 : Gain  Gain=1715  SaturateOnIntegerOverflow=on  OutDataTypeStr=Inherit: Same as input  ParamDataTypeStr=Inherit: Same as input
  rho0 : Gain  Gain=2.377e-3  SaturateOnIntegerOverflow=on  OutDataTypeStr=Inherit: Same as input  ParamDataTypeStr=Inherit: Same as input
  qbar / ps : Outport  VectorParamsAs1DForOutWhenUnconnected=off
  wires:
  h (ft)/1 -> r2d2/1, Switch/2
  Sum3/1 -> Math Function/1, r2d3/1  "tfac"
  Constant3/1 -> Switch/1
  r2d3/1 -> Switch/3
  Constant6/1 -> Math Function/2
  rho0/1 -> Product5/1, Product6/2  "rho"
  r2d2/1 -> Sum3/2
  Constant2/1 -> Sum3/1
  Math Function/1 -> rho0/1
  Math Function1/1 -> Product5/2
  Switch/1 -> r2d5/1  "temp"
  r2d5/1 -> Product6/1
  Product6/1 -> Product/1  "ps"
  Product5/1 -> r2d4/1  "qbar"
  Product/1 -> qbar / ps/1
  Vt (ft/s)/1 -> Math Function1/1  "Vt (ft/s)"
  r2d4/1 -> Product/2

== system Linearization/Aerodynamic1/ISP  ==
  note: 1 T
      | 2 a (Speed of sound)
      | 3 P
      | 4 rho
      | 5 g
      | 6 mu (Coefficient of viscosity)
  h (ft) : Inport
  Vt (ft/s) : Inport  Port=2
  Demux : Demux  Outputs=[1,1,1,1,1,1]
      settings: DisplayOption=none
  Divide1 : Product  Inputs=*/
  Length Conversion : aerolibconvert2/Length Conversion  IU=ft  OU=m
  MATLAB Function : MATLAB Function  TreatAsAtomicUnit=on
  Product : Product
  Square : Math  Operator=square  SignedPower=on
  To Workspace : ToWorkspace  VariableName=mach  SaveFormat=Timeseries  SampleTime=-1
  r2d1 : Gain  Gain=0.5  SaturateOnIntegerOverflow=on  OutDataTypeStr=Inherit: Same as input  ParamDataTypeStr=Inherit: Same as input
  r2d3 : Gain  Gain=3.2808399  SaturateOnIntegerOverflow=on  OutDataTypeStr=Inherit: Same as input  ParamDataTypeStr=Inherit: Same as input
  r2d4 : Gain  Gain=0.00194032033  SaturateOnIntegerOverflow=on  OutDataTypeStr=Inherit: Same as input  ParamDataTypeStr=Inherit: Same as input
  T(K) : Outport  VectorParamsAs1DForOutWhenUnconnected=off
  "Mach " : Outport  Port=2  VectorParamsAs1DForOutWhenUnconnected=off
  P(HPa) : Outport  Port=3  VectorParamsAs1DForOutWhenUnconnected=off
  "qbar " : Outport  Port=4  VectorParamsAs1DForOutWhenUnconnected=off
  rho : Outport  Port=5  VectorParamsAs1DForOutWhenUnconnected=off
  g (m/s^2) : Outport  Port=6  VectorParamsAs1DForOutWhenUnconnected=off
  mu : Outport  Port=7  VectorParamsAs1DForOutWhenUnconnected=off
  wires:
  r2d3/1 -> Divide1/2
  r2d1/1 -> Product/2
  Demux/4 -> rho/1, r2d4/1  "rho(kg/m^3)"
  Demux/2 -> r2d3/1  "a(m/s)"
  Demux/1 -> T(K)/1  "T(K)"
  r2d4/1 -> r2d1/1
  Divide1/1 -> To Workspace/1, "Mach "/1
  Demux/5 -> g (m/s^2)/1  "g (m/s^2)"
  Demux/6 -> mu/1  "mu"
  Product/1 -> "qbar "/1
  Square/1 -> Product/1
  Vt (ft/s)/1 -> Square/1, Divide1/1
  Demux/3 -> P(HPa)/1  "P(Pa)"
  h (ft)/1 -> Length Conversion/1
  Length Conversion/1 -> MATLAB Function/1(h)
  MATLAB Function/1(ISP_output) -> Demux/1

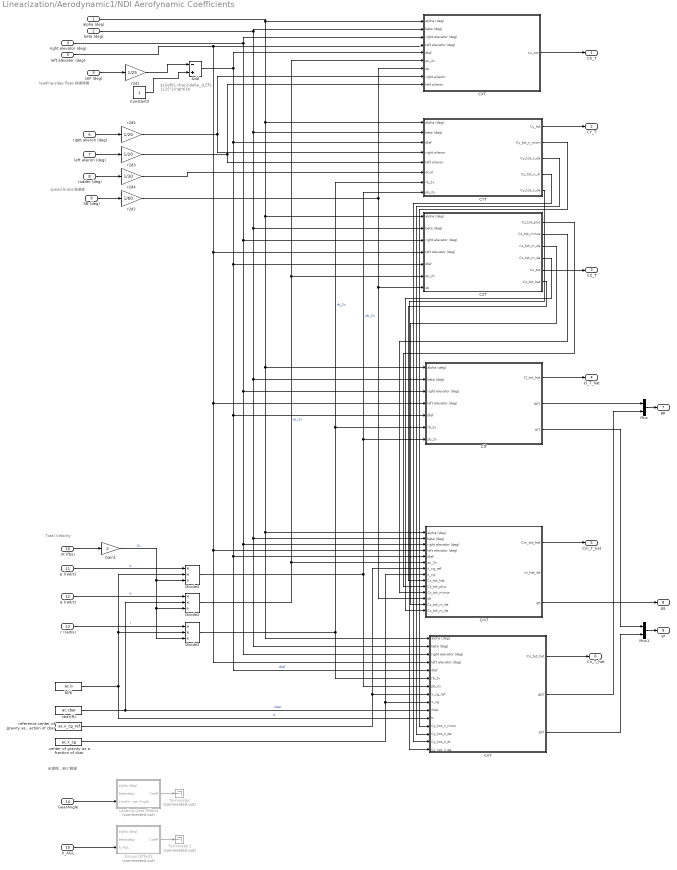
== system Linearization/Aerodynamic1/NDI Aerofynamic Coefficients ==
  note: leading-edge flaps
      | 前緣襟翼
  note: speed brake
      | 減速板
  note: Total Velocity
  note: 未建模，缺少數據
  note: ${\left(1-\frac{\delta_{LEF} }{25°}\right)}$
  alpha (deg) : Inport
  beta (deg) : Inport  Port=2
  LEF (deg) : Inport  Port=3
  right elevator (deg) : Inport  Port=4
  left elevator (deg) : Inport  Port=5
  right alieron (deg) : Inport  Port=6
  left alieron (deg) : Inport  Port=7
  rudder (deg) : Inport  Port=8
  SB (deg) : Inport  Port=9  Unit=deg
  Vt (ft/s) : Inport  Port=10
  p (rad/s) : Inport  Port=11
  q (rad/s) : Inport  Port=12
  r (rad/s) : Inport  Port=13
  GearAngle : Inport  Port=14
  h_AGL : Inport  Port=15
  Add : Sum  Inputs=-+
  CXT : Subsystem
  CYT : Subsystem
  CZT : Subsystem
  ClT : Subsystem
  CmT : Subsystem
  CnT : Subsystem
  Constant3 : Constant
  Divide2 : Product  Inputs=**/
  Divide3 : Product  Inputs=**/
  Divide4 : Product  Inputs=**/
  Gain1 : Gain  Gain=2
  Ground Effects : Subsystem  Commented=on
  Landing Gear Effects : Subsystem  Commented=on
  Mux : Mux  Inputs=2
  Mux1 : Mux  Inputs=2
  Terminator : Terminator  Commented=on
  Terminator1 : Terminator  Commented=on
  b(ft) : Constant  Value=ac.b
  cbar(ft) : Constant  Value=ac.cbar
  center of gravity as a fraction of cbar : Constant  Value=ac.x_cg
  r2d1 : Gain  Gain=1/25  SaturateOnIntegerOverflow=on  OutDataTypeStr=Inherit: Same as input  ParamDataTypeStr=Inherit: Same as input
  r2d2 : Gain  Gain=1/60  SaturateOnIntegerOverflow=on  OutDataTypeStr=Inherit: Same as input  ParamDataTypeStr=Inherit: Same as input
  r2d3 : Gain  Gain=1/20  SaturateOnIntegerOverflow=on  OutDataTypeStr=Inherit: Same as input  ParamDataTypeStr=Inherit: Same as input
  r2d4 : Gain  Gain=1/30  SaturateOnIntegerOverflow=on  OutDataTypeStr=Inherit: Same as input  ParamDataTypeStr=Inherit: Same as input
  r2d5 : Gain  Gain=1/20  SaturateOnIntegerOverflow=on  OutDataTypeStr=Inherit: Same as input  ParamDataTypeStr=Inherit: Same as input
  reference center of gravity as a fraction of cbar : Constant  Value=ac.x_cg_ref
  CX_T : Outport  VectorParamsAs1DForOutWhenUnconnected=off
  CY_T : Outport  Port=2  VectorParamsAs1DForOutWhenUnconnected=off
  CZ_T : Outport  Port=3  VectorParamsAs1DForOutWhenUnconnected=off
  Cl_T_hat : Outport  Port=4  VectorParamsAs1DForOutWhenUnconnected=off
  Cm_T_hat : Outport  Port=5  VectorParamsAs1DForOutWhenUnconnected=off
  Cn_T_hat : Outport  Port=6  VectorParamsAs1DForOutWhenUnconnected=off
  gp : Outport  Port=7  VectorParamsAs1DForOutWhenUnconnected=off
  gq : Outport  Port=8  VectorParamsAs1DForOutWhenUnconnected=off
  gr : Outport  Port=9  VectorParamsAs1DForOutWhenUnconnected=off
  wires:
  alpha (deg)/1 -> CXT/1(alpha (deg)), CnT/1(alpha (deg)), CmT/1(alpha (deg)), ClT/1(alpha (deg)), CZT/1(alpha (deg)), CYT/1(alpha (deg))
  beta (deg)/1 -> CXT/2(beta (deg)), CnT/2(beta (deg)), CmT/2(beta (deg)), ClT/2(beta (deg)), CZT/2(beta (deg)), CYT/2(beta (deg))
  right elevator (deg)/1 -> CXT/3(right elevator (deg)), CnT/3(right elevator (deg)), CmT/3(right elevator (deg)), ClT/3(right elevator (deg)), CZT/3(right elevator (deg))
  Vt (ft/s)/1 -> Gain1/1
  p (rad/s)/1 -> Divide4/1  "p"
  q (rad/s)/1 -> Divide2/1  "q"
  r (rad/s)/1 -> Divide3/1  "r"
  b(ft)/1 -> Divide4/2, Divide3/2, CnT/11(b)  "b"
  cbar(ft)/1 -> Divide2/2, CnT/10(cbar)  "cbar"
  Add/1 -> CXT/5(dlef), CnT/5(dlef), CmT/5(dlef), ClT/5(dlef), CZT/5(dlef), CYT/3(dlef)  "dlef"
  left alieron (deg)/1 -> r2d3/1
  rudder (deg)/1 -> r2d4/1
  Divide2/1 -> CXT/6(qc_2v), CZT/6(qc_2v), CmT/6(qc_2v)  "qc_2v"
  r2d4/1 -> CYT/6(drud)
  Divide3/1 -> CnT/6(rb_2v), CYT/7(rb_2v), ClT/6(rb_2v)  "rb_2v"
  Divide4/1 -> CnT/7(pb_2v), CYT/8(pb_2v), ClT/7(pb_2v)  "pb_2v"
  reference center of gravity as a fraction of cbar/1 -> CmT/7(x_cg_ref), CnT/8(x_cg_ref)
  center of gravity as a fraction of cbar/1 -> CmT/8(x_cg), CnT/9(x_cg)
  CZT/1(Cz_tot_plus) -> CmT/10(Cz_tot_plus)
  CZT/2(Cz_tot_minus) -> CmT/11(Cz_tot_minus)
  CYT/2(Cy_tot_n_mom) -> CnT/12(Cy_tot_n_mom)
  CYT/3(Cy_tot_n_da) -> CnT/13(Cy_tot_n_da)
  CYT/4(Cy_tot_n_dr) -> CnT/14(Cy_tot_n_dr)
  SB (deg)/1 -> r2d2/1
  CXT/1(Cx_tot) -> CX_T/1
  CYT/1(Cy_tot) -> CY_T/1
  CZT/5(Cz_tot) -> CZ_T/1
  CnT/1(Cn_tot_hat) -> Cn_T_hat/1
  CmT/1(Cm_tot_hat) -> Cm_T_hat/1
  ClT/1(Cl_tot_hat) -> Cl_T_hat/1
  LEF (deg)/1 -> r2d1/1
  r2d2/1 -> CXT/7(sb), CmT/12(sb), CZT/7(sb)
  Gain1/1 -> Divide3/3, Divide2/3, Divide4/3  "2v"
  Landing Gear Effects/1(Coeff) -> Terminator/1
  h_AGL/1 -> Ground Effects/3(h_AGL)
  Ground Effects/1(Coeff) -> Terminator1/1
  GearAngle/1 -> Landing Gear Effects/3(Landing Gear Angle)
  right alieron (deg)/1 -> r2d5/1
  r2d5/1 -> CXT/8(right aileron), CYT/4(right aileron)
  r2d3/1 -> CYT/5(left aileron), CXT/9(left aileron)
  r2d1/1 -> Add/1
  Constant3/1 -> Add/2
  left elevator (deg)/1 -> CXT/4(left elevator (deg)), CnT/4(left elevator (deg)), CmT/4(left elevator (deg)), ClT/4(left elevator (deg)), CZT/4(left elevator (deg))
  Mux1/1 -> gr/1
  CmT/3(gq) -> gq/1
  CnT/3(gr2) -> Mux1/2
  ClT/3(gr1) -> Mux1/1
  CnT/2(gp2) -> Mux/2
  Mux/1 -> gp/1
  ClT/2(gp1) -> Mux/1
  CZT/6(Cz_tot_hat) -> CmT/9(Cz_tot_hat)
  CYT/5(Cy_tot_n_de) -> CnT/15(Cy_tot_n_de)
  CZT/3(Cz_tot_m_de) -> CmT/13(Cz_tot_m_de)
  CZT/4(Cz_tot_m_da) -> CmT/14(Cz_tot_m_da)

== system Linearization/Environment1/Dynamic Pressure ==
  Vt : Inport
  rho : Inport  Port=2
  1/2rhoV^2 : Gain  Gain=1/2  SaturateOnIntegerOverflow=on  OutDataTypeStr=Inherit: Same as input  ParamDataTypeStr=Inherit: Same as input
  Product2 : Product  InputSameDT=on  SaturateOnIntegerOverflow=on  OutDataTypeStr=Inherit: Same as first input
  Square : Math  Operator=square  SignedPower=on
  qbar : Outport
  wires:
  rho/1 -> Product2/2
  Square/1 -> Product2/1
  1/2rhoV^2/1 -> qbar/1
  Product2/1 -> 1/2rhoV^2/1
  Vt/1 -> Square/1

== system Linearization/Environment1/ISP  ==
  note: 1 T
      | 2 a (Speed of sound)
      | 3 P
      | 4 rho
      | 5 g
      | 6 mu (Coefficient of viscosity)
  h(m) : Inport
  Demux : Demux  Outputs=[1,1,1,1,1,1]
      settings: DisplayOption=none
  MATLAB Function : MATLAB Function  TreatAsAtomicUnit=on
  end8 : Terminator
  end9 : Terminator
  T (K) : Outport  VectorParamsAs1DForOutWhenUnconnected=off
  a (m/s) : Outport  Port=2  VectorParamsAs1DForOutWhenUnconnected=off
  P (HPa) : Outport  Port=3  VectorParamsAs1DForOutWhenUnconnected=off
  rho (kg/m^3) : Outport  Port=4  VectorParamsAs1DForOutWhenUnconnected=off
  wires:
  MATLAB Function/1(ISP_output) -> Demux/1
  h(m)/1 -> MATLAB Function/1(h)
  Demux/4 -> rho (kg/m^3)/1  "rho(kg/m^3)"
  Demux/2 -> a (m/s)/1  "a(m/s)"
  Demux/1 -> T (K)/1  "T(K)"
  Demux/5 -> end8/1  "g (m/s^2)"
  Demux/6 -> end9/1  "mu"
  Demux/3 -> P (HPa)/1  "P(Pa)"

== system Linearization/Environment1/Mach Number ==
  Vt : Inport
  a : Inport  Port=2
  Product1 : Product  Inputs=*/  InputSameDT=on  SaturateOnIntegerOverflow=on  OutDataTypeStr=Inherit: Same as first input
  Mach : Outport  Unit=1  VectorParamsAs1DForOutWhenUnconnected=off
  wires:
  Vt/1 -> Product1/1
  a/1 -> Product1/2
  Product1/1 -> Mach/1

== system Linearization/Rotation Speed(TVC OFF)OK/If Action Subsystem ==
  pqr command : Inport
  Action Port : ActionPort  ActionPortLabel=if( u1 > 220)
  Out1 : Outport
  wires:
  pqr command/1 -> Out1/1

== system Linearization/Rotation Speed(TVC OFF)OK/If Action Subsystem1 ==
  In1 : Inport
  Action Port : ActionPort  ActionPortLabel=elseif(220 >= u1 >= 135)
  Mux1 : Mux  Inputs=3
  Out1 : Outport
  wires:
  In1/1 -> Mux1/3, Mux1/1, Mux1/2
  Mux1/1 -> Out1/1  "pqr dot desire"
